simulink library "aerolib3dof"  (Simulink 5.0)
libraries: aerolibutil x2, simulink x2
settings Model: Creator=sgage  LastModifiedBy=sgage  ExtModeAutoUpdateStatusClock=off  TargetHWChar=2  TargetHWWordLengths=8,16,32,32
settings Model: ForwardingTableString=|
  | ||__slOldName__||aerolib3dof/ Equations of Motion
  | (Body Axes)||__slNewName__||aerolibprivatev1p5/3DoF (Body Axes)||__slOldName__||aerolib3dof/Incidence
  | & Airspeed||__slNewName__||aerolibasang/Incidence
  | & Airspeed

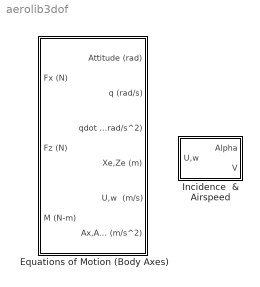
== system aerolib3dof ==
  " Equations of Motion (Body Axes)" : Subsystem  mask(3DoF EoM){v_ini=100, theta_ini=0, alpha_ini=0, q_ini=0, pos_ini=[0 0], mass=1, Iyy=1, g=9.81}
      mask prompts: v_ini "Initial velocity [m/s]:"; theta_ini "Initial body attitude [rad]:"; alpha_ini "Initial incidence [rad]:"; q_ini "Initial body rotation rate [rad/sec]:"; pos_ini "Initial position (x z) [m]:"; mass "Mass [Kg]:"; Iyy "Inertia [Kg.m^2]:"; g "Acceleration due to gravity [m/s/s]:"
      mask help:
      | Integrate the three-degrees-of-freedom equations of motion to determine body position, velocity, attitude, and related values.
      |
      | Inputs are forces on the body in x-axis, forces on the body in z-axis, and moments on the body along y-axis.  Outputs are pitch angle, pitch rate, pitch acceleration, position in x-axis and z-axis in Earth coordinates, translational velocity in x-axis and z-axis, and acceleration in x-axis and z-axis due to body forces.
      mask init:
      | U0 = v_ini*cos(alpha_ini);
      | w0 = v_ini*sin(alpha_ini);
      mask Help: web(asbhelp('equationsofmotion'));
  Incidence  & Airspeed : Subsystem
      mask Type: Incidence&Airspeed
      mask Description: Calculate the angle between the body and the velocity vector (incidence) and the velocity magnitude from the components in body axes (U,w).
      mask Help: web(asbhelp);

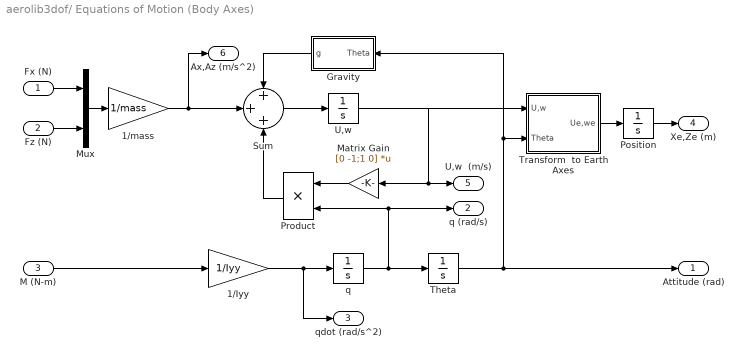
== system aerolib3dof/ Equations of Motion (Body Axes) ==
  Fx (N) : Inport  ShowAdditionalParam=on  DataType=double
  Fz (N) : Inport  Port=2  ShowAdditionalParam=on  DataType=double
  M (N-m) : Inport  Port=3  ShowAdditionalParam=on  DataType=double
  1/Iyy : Gain  Gain=1/Iyy  SaturateOnIntegerOverflow=on
  1/mass : Gain  Gain=1/mass  SaturateOnIntegerOverflow=on
  Gravity : Subsystem  Orientation=left
  Matrix Gain : Gain  Orientation=left  Gain=[0 -1;1 0]  Multiplication=Matrix(K*u)  SaturateOnIntegerOverflow=on
  Mux : Mux  Inputs=2
  Position : Integrator  InitialCondition=pos_ini
  Product : Product  Orientation=left  SaturateOnIntegerOverflow=on  InputSameDT=on
  Sum : Sum  Inputs=+++  SaturateOnIntegerOverflow=on  InputSameDT=on
  Theta : Integrator  InitialCondition=theta_ini
  Transform  to Earth Axes : Subsystem
  U,w : Integrator  InitialCondition=[U0 w0]
  q : Integrator  InitialCondition=q_ini
  Attitude (rad) : Outport  InitialOutput=0
  q (rad/s) : Outport  Port=2  InitialOutput=0
  qdot (rad/s^2) : Outport  Port=3  InitialOutput=0
  Xe,Ze (m) : Outport  Port=4  InitialOutput=0
  "U,w  (m/s) " : Outport  Port=5  InitialOutput=0
  Ax,Az (m/s^2) : Outport  Port=6  InitialOutput=0
  wires:
  Gravity/1(g) -> Sum/1
  1/mass/1 -> Sum/2, Ax,Az (m/s^2)/1
  Product/1 -> Sum/3
  Mux/1 -> 1/mass/1
  Fz (N)/1 -> Mux/2
  Fx (N)/1 -> Mux/1
  Transform  to Earth Axes/1(Ue,we) -> Position/1
  Matrix Gain/1 -> Product/1
  Position/1 -> Xe,Ze (m)/1
  U,w/1 -> "U,w  (m/s) "/1, Transform  to Earth Axes/1(U,w), Matrix Gain/1
  Theta/1 -> Gravity/1(Theta), Transform  to Earth Axes/2(Theta), Attitude (rad)/1
  1/Iyy/1 -> qdot (rad/s^2)/1, q/1
  M (N-m)/1 -> 1/Iyy/1
  q/1 -> Product/2, q (rad/s)/1, Theta/1
  Sum/1 -> U,w/1

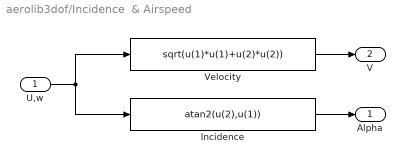
== system aerolib3dof/Incidence  & Airspeed ==
  U,w : Inport
  Incidence : Fcn  Expr=atan2(u(2),u(1))
  Velocity : Fcn  Expr=sqrt(u(1)*u(1)+u(2)*u(2))
  Alpha : Outport  InitialOutput=0
  V : Outport  Port=2  InitialOutput=0
  wires:
  U,w/1 -> Incidence/1, Velocity/1
  Incidence/1 -> Alpha/1
  Velocity/1 -> V/1

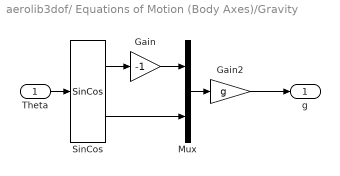
== system aerolib3dof/ Equations of Motion (Body Axes)/Gravity ==
  Theta : Inport
  Gain : Gain  Gain=-1  SaturateOnIntegerOverflow=on
  Gain2 : Gain  Gain=g  SaturateOnIntegerOverflow=on
  Mux : Mux  Inputs=2
  SinCos : aerolibutil/SinCos
  g : Outport
  wires:
  Gain2/1 -> g/1
  Mux/1 -> Gain2/1
  SinCos/2 -> Mux/2
  Gain/1 -> Mux/1
  SinCos/1 -> Gain/1
  Theta/1 -> SinCos/1

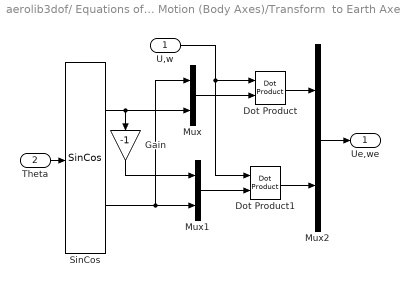
== system aerolib3dof/ Equations of Motion (Body Axes)/Transform  to Earth Axes ==
  U,w : Inport
  Theta : Inport  Port=2
  Dot Product : simulink/Math Operations/Dot Product  OutDataType=sfix(16)  OutScaling=2^-10  DoSatur=on
  Dot Product1 : simulink/Math Operations/Dot Product  OutDataType=sfix(16)  OutScaling=2^-10  DoSatur=on
  Gain : Gain  Orientation=down  Gain=-1  SaturateOnIntegerOverflow=on
  Mux : Mux  Inputs=2
  Mux1 : Mux  Inputs=2
  Mux2 : Mux  Inputs=2
  SinCos : aerolibutil/SinCos
  Ue,we : Outport
  wires:
  Gain/1 -> Mux1/1
  SinCos/1 -> Mux/2, Gain/1
  U,w/1 -> Dot Product1/1, Dot Product/1
  Mux/1 -> Dot Product/2
  Mux2/1 -> Ue,we/1
  Dot Product1/1 -> Mux2/2
  Dot Product/1 -> Mux2/1
  Mux1/1 -> Dot Product1/2
  SinCos/2 -> Mux1/2, Mux/1
  Theta/1 -> SinCos/1
